simulink model "Num2BD"  (R2023b)
settings: Solver=FixedStepAuto  StartTime=0.0  StopTime=10.0  FixedStep=0.5  RelTol=1e-3
settings Model: Creator=lyndo  LastModifiedBy=lyndo

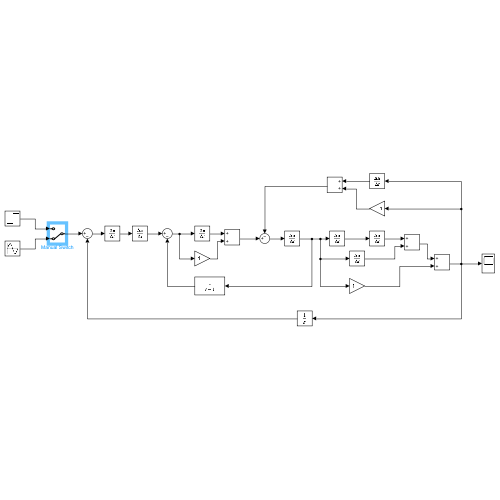
[thumbnail: Simulink's stored preview of the top-level diagram]
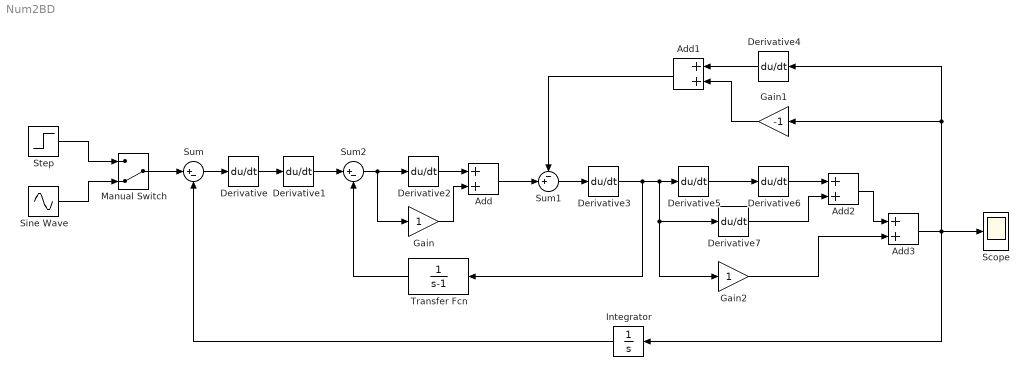
== system Num2BD ==
  Add{,1..3} (4 alike) : Sum
  Derivative{,1..7} (8 alike) : Derivative
  Gain : Gain
  Gain1 : Gain  Gain=-1
  Gain2 : Gain
  Integrator : Integrator
  Manual Switch : ManualSwitch  CurrentSetting=0
  Scope : Scope
  Sine Wave : Sin  SampleTime=0
  Step : Step  SampleTime=0
  Sum : Sum  Inputs=|+-
  Sum1 : Sum  Inputs=-+|
  Sum2 : Sum  Inputs=|+-
  Transfer Fcn : TransferFcn  Denominator=[1 -1]
  wires:
  Sine Wave/1 -> Manual Switch/2
  Step/1 -> Manual Switch/1
  Derivative/1 -> Derivative1/1
  Manual Switch/1 -> Sum/1
  Sum/1 -> Derivative/1
  Derivative1/1 -> Sum2/1
  Sum2/1 -> Gain/1, Derivative2/1
  Gain/1 -> Add/2
  Derivative2/1 -> Add/1
  Add/1 -> Sum1/2
  Sum1/1 -> Derivative3/1
  Derivative3/1 -> Transfer Fcn/1, Gain2/1, Derivative7/1, Derivative5/1
  Transfer Fcn/1 -> Sum2/2
  Derivative4/1 -> Add1/1
  Gain1/1 -> Add1/2
  Derivative5/1 -> Derivative6/1
  Add2/1 -> Add3/1
  Derivative6/1 -> Add2/1
  Derivative7/1 -> Add2/2
  Gain2/1 -> Add3/2
  Add3/1 -> Scope/1, Derivative4/1, Gain1/1, Integrator/1
  Integrator/1 -> Sum/2
  Add1/1 -> Sum1/1
